simulink model "test"  (R2018b)
settings: Solver=VariableStepAuto  StartTime=0.0  StopTime=5  RelTol=1e-3
values from neighbouring files (symbols this model uses):
  Den = cell2mat(G_model.Denominator)    [test.m]
  Kden = cell2mat(K.Denominator)    [test.m]
  KNum = cell2mat(K.Numerator)    [test.m]
  Num = cell2mat(G_model.Numerator)    [test.m]
  Pden = cell2mat(P_trap.Denominator)    [test.m]
  PNum = cell2mat(P_trap.Numerator)    [test.m]
settings Model: Creator=57531  LastModifiedBy=57531

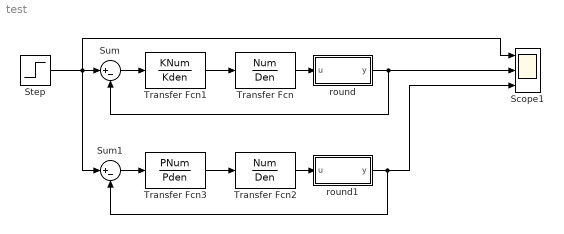
== system test ==
  Scope1 : Scope  NumInputPorts=3
  Step : Step  Time=0.2  SampleTime=0
  Sum : Sum  Inputs=|+-
  Sum1 : Sum  Inputs=|+-
  Transfer Fcn : TransferFcn  Numerator=Num  Denominator=Den
  Transfer Fcn1 : TransferFcn  Numerator=KNum  Denominator=Kden
  Transfer Fcn2 : TransferFcn  Numerator=Num  Denominator=Den
  Transfer Fcn3 : TransferFcn  Numerator=PNum  Denominator=Pden
  round : MATLAB Function  TreatAsAtomicUnit=on
  round1 : MATLAB Function  TreatAsAtomicUnit=on
  wires:
  Transfer Fcn1/1 -> Transfer Fcn/1
  Sum/1 -> Transfer Fcn1/1
  Sum1/1 -> Transfer Fcn3/1
  Transfer Fcn3/1 -> Transfer Fcn2/1
  Transfer Fcn/1 -> round/1(u)
  Transfer Fcn2/1 -> round1/1(u)
  Step/1 -> Scope1/1, Sum1/1, Sum/1
  round/1(y) -> Sum/2, Scope1/2
  round1/1(y) -> Scope1/3, Sum1/2

== matlab function test/round1 ==
  data: u input; y output
function y = fcn(u)
y = round(u * 50000) / 50000;

== matlab function test/round ==
  data: u input; y output
function y = fcn(u)
y = round(u * 50000) / 50000;
